simulink model "thrust_observer"  (R2017a)
settings: Solver=VariableStepAuto  StartTime=0.0  StopTime=2  MaxStep=1e-3  RelTol=1e-3
values from neighbouring files (symbols this model uses):
  A = [0 1 ... (first row only)    [system_id.m]    (also in thrust_control_data.m)
  Ad = [Ad ... (first row only)    [thrust_control_data.m]
  B = [0 ... (first row only)    [system_id.m]    (also in thrust_control_data.m)
  Bd = [zeros(n+l-1, 1) ... (first row only)    [thrust_control_data.m]
  C = [1 0]    [system_id.m]    (also in thrust_control_data.m)
  H = acker(A', C', [-5 -5])'    [thrust_control_data.m]
  Hd = acker(Aobs', Cobs', 0.4 * ones(1, n+l+1))'    [thrust_control_data.m]
  T = 1/30    (= 0.0333333333333)    [drone_data_process.m]    (also in thrust_control_data.m)
settings Model: Creator=sdc  LastModifiedBy=sdc

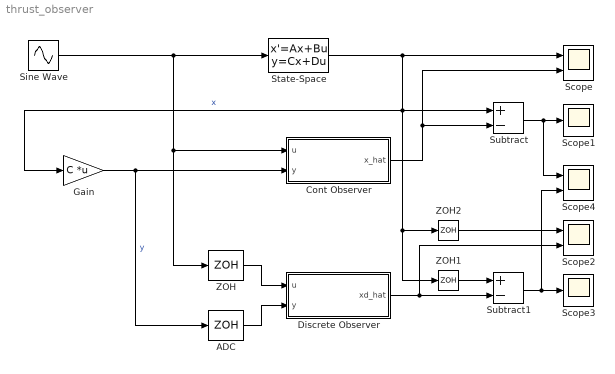
== system thrust_observer ==
  ADC : ZeroOrderHold  SampleTime=T
  Cont Observer : Subsystem
  Discrete Observer : Subsystem
  Gain : Gain  Gain=C  Multiplication=Matrix(K*u)
  Scope : Scope  NumInputPorts=2
  Scope1 : Scope
  Scope2 : Scope  NumInputPorts=2
  Scope3 : Scope
  Scope4 : Scope  NumInputPorts=2
  Sine Wave : Sin  Amplitude=500  SampleTime=0
  State-Space : StateSpace  A=A  B=B  C=eye(2)  D=zeros(2,1)  X0=[1;0.1]
  Subtract : Sum  Inputs=+-
  Subtract1 : Sum  Inputs=+-
  ZOH : ZeroOrderHold  SampleTime=T
  ZOH1 : ZeroOrderHold  SampleTime=T
  ZOH2 : ZeroOrderHold  SampleTime=T
  wires:
  Sine Wave/1 -> ZOH/1, Cont Observer/1(u), State-Space/1
  State-Space/1 -> Gain/1, ZOH1/1, ZOH2/1, Subtract/1, Scope/1  "x"
  Cont Observer/1("x_hat ") -> Subtract/2, Scope/2
  Gain/1 -> ADC/1, Cont Observer/2(y)  "y"
  Subtract/1 -> Scope4/1, Scope1/1
  ZOH/1 -> Discrete Observer/1(u)
  ADC/1 -> Discrete Observer/2(y)
  Discrete Observer/1(xd_hat) -> Subtract1/2, Scope2/2
  Subtract1/1 -> Scope4/2, Scope3/1
  ZOH1/1 -> Subtract1/1
  ZOH2/1 -> Scope2/1

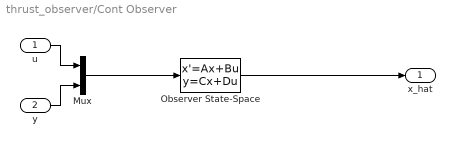
== system thrust_observer/Cont Observer ==
  u : Inport
  y : Inport  Port=2
  Mux : Mux  Inputs=2
  Observer State-Space : StateSpace  A=A-H*C  B=[B,H]  C=eye(2)  D=zeros(2,2)  X0=0
  "x_hat " : Outport
  wires:
  u/1 -> Mux/1
  y/1 -> Mux/2
  Mux/1 -> Observer State-Space/1
  Observer State-Space/1 -> "x_hat "/1

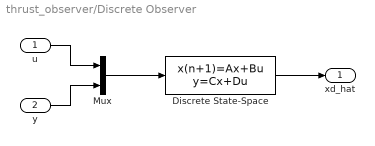
== system thrust_observer/Discrete Observer ==
  u : Inport
  y : Inport  Port=2
  Discrete State-Space : DiscreteStateSpace  A=Ad-Hd*C  B=[Bd, Hd]  C=eye(2)  D=zeros(2,2)  SampleTime=T
  Mux : Mux  Inputs=2
  xd_hat : Outport
  wires:
  u/1 -> Mux/1
  y/1 -> Mux/2
  Mux/1 -> Discrete State-Space/1
  Discrete State-Space/1 -> xd_hat/1
